simulink model "PILnewH"  (R2021a)
settings: Solver=FixedStepAuto  StartTime=0.0  StopTime=41.24  FixedStep=0.001  RelTol=1e-3  EnableMultiTasking=on
values from neighbouring files (symbols this model uses):
  den_lpf_d = den_lpf20    [Mainframe_init.m]    (also in load_autopilot.m)
  Emulated_FCC_IO_Delay = 7    [Mainframe_init.m]
  Enable_Gyros = 0    [Mainframe_init.m]
  Enable_INS = 0    [Mainframe_init.m]
  num_lpf_d = num_lpf20    [Mainframe_init.m]    (also in load_autopilot.m)
undefined symbols (not defined in the file or in its folder): act_dmp, act_omega, Actuator, Aerodynamics, aMode, Autopilot, AUX, c_b_WGS, c_be, c_flat, c_grav, c_h_geop0, c_h_geope, c_pa0, c_pe, c_r0, c_rot, c_rsma, c_Tmp0, d_siB_0, d_siB_max, d_siB_min, dd_siB_max, dd_siB_min, dev, DiscIntNeverNeededParam, e_pa, e_Tmp, Earth, fin_maxrate, flag_I_act_switch, flag_I_aero_switch, flag_I_flat, flag_I_gravity_switch, flag_I_rot, hcr, HIL_Data, JMMM_0, JMMM_e, JSPB_e, lat_0, lon_0, Mass_Props, mB_0, mM_0, mM_e, National_Instruments, pBII_0, PCIe, pMPB, pNPB, propellant_kg, prp_FBPB, prp_mdot, prp_T, pSPB, pwm_output1, qEG_0, qIB_0, qIE_0 ... (+29)
libraries: simulink x31, simulink_extras x24, aerolibcommonsys x4, px4lib x2, custom_blocks x1, pil_lib x1, aerolibtransform2 x1, sldrtlib x1, aerolibnav x1
(part 5 of 15)

== system PILnewH/Non-linear Flight Dynamic Model/GRM_Airframe/motion_kinematics/calc_motion_kinematics/earth_rotation ==
  lat : Inport
  lon : Inport  Port=2
  Gain : Gain
  Gain1 : Gain
  earth_rotation_rate : Subsystem
  quaternion_integration : Subsystem
  quaternion_integration1 : Subsystem
  transport_rate : Subsystem
  wIEE : Outport  VectorParamsAs1DForOutWhenUnconnected=off
  TIE : Outport  Port=2  VectorParamsAs1DForOutWhenUnconnected=off
  qIE : Outport  Port=3  VectorParamsAs1DForOutWhenUnconnected=off
  qEG : Outport  Port=4  VectorParamsAs1DForOutWhenUnconnected=off
  TEG : Outport  Port=5  VectorParamsAs1DForOutWhenUnconnected=off
  wEGG : Outport  Port=6  VectorParamsAs1DForOutWhenUnconnected=off
  wires:
  earth_rotation_rate/1(wIEE) -> wIEE/1, Gain/1
  Gain/1 -> quaternion_integration/1(wEIE)  "wEIE"
  quaternion_integration/1(qIE) -> qIE/1
  quaternion_integration/2(TIE) -> TIE/1
  lat/1 -> transport_rate/1(lat)
  lon/1 -> transport_rate/2(lon)
  transport_rate/1(wEGG) -> wEGG/1, Gain1/1
  Gain1/1 -> quaternion_integration1/1(wGEG)  "wGEG"
  quaternion_integration1/1(qEG) -> qEG/1
  quaternion_integration1/2(TEG) -> TEG/1

== system PILnewH/Non-linear Flight Dynamic Model/GRM_Airframe/propulsion/prp_uncertainty/3_rot_mat ==
  wi1 : Inport
  wi2 : Inport  Port=2
  wi3 : Inport  Port=3
  1. Rotation x-Achse : Subsystem
  1. Rotation y-Achse : Subsystem
  1. Rotation z-Achse : Subsystem
  2. Rotation x-Achse : Subsystem
  2. Rotation y-Achse : Subsystem
  2. Rotation z-Achse : Subsystem
  3. Rotation : Product  Inputs=***  Multiplication=Matrix(*)
  3. Rotation x-Achse : Subsystem
  3. Rotation y-Achse : Subsystem
  3. Rotation z-Achse : Subsystem
  Constant : Constant  Value=rot_1
  Constant1 : Constant  Value=rot_2
  Constant2 : Constant  Value=rot_3
  Multiport Switch : MultiPortSwitch
  Multiport Switch1 : MultiPortSwitch
  Multiport Switch2 : MultiPortSwitch
  T12 : Outport  VectorParamsAs1DForOutWhenUnconnected=off
  wires:
  Multiport Switch2/1 -> 3. Rotation/1
  Multiport Switch1/1 -> 3. Rotation/2
  Multiport Switch/1 -> 3. Rotation/3
  wi3/1 -> 3. Rotation x-Achse/1(alpha3), 3. Rotation z-Achse/1(alpha3), 3. Rotation y-Achse/1(alpha3)
  wi1/1 -> 1. Rotation z-Achse/1(alpha1), 1. Rotation y-Achse/1(alpha1), 1. Rotation x-Achse/1(alpha1)
  wi2/1 -> 2. Rotation z-Achse/1(alpha2), 2. Rotation y-Achse/1(alpha2), 2. Rotation x-Achse/1(alpha2)
  3. Rotation z-Achse/1(3Rot_Matrix_z) -> Multiport Switch2/4
  Constant/1 -> Multiport Switch/1
  1. Rotation x-Achse/1(1Rot_Matrix_x) -> Multiport Switch/2
  Constant1/1 -> Multiport Switch1/1
  1. Rotation y-Achse/1(1Rot_Matrix_y) -> Multiport Switch/3
  1. Rotation z-Achse/1(1Rot_Matrix_z) -> Multiport Switch/4
  Constant2/1 -> Multiport Switch2/1
  3. Rotation/1 -> T12/1  "T12"
  2. Rotation x-Achse/1(2Rot_Matrix_x) -> Multiport Switch1/2
  2. Rotation y-Achse/1(2Rot_Matrix_y) -> Multiport Switch1/3
  2. Rotation z-Achse/1(2Rot_Matrix_z) -> Multiport Switch1/4
  3. Rotation y-Achse/1(3Rot_Matrix_y) -> Multiport Switch2/3
  3. Rotation x-Achse/1(3Rot_Matrix_x) -> Multiport Switch2/2

== system PILnewH/Non-linear Flight Dynamic Model/GRM_Airframe/propulsion/prp_uncertainty/cross_product ==
  note: Outputs [size]:
      |
      | r1 x r2  [3x1]
  note: Inputs [size]:
      |
      | r1 [3x1]
      | r2 [3x1]
  r1 : Inport
  r2 : Inport  Port=2
  Demux2 : Demux  Outputs=[1;1;1]
      settings: DisplayOption=none
  Demux3 : Demux  Outputs=[1;1;1]
      settings: DisplayOption=none
  Product{2..7} (6 alike) : Product  InputSameDT=on  RndMeth=Zero  SaturateOnIntegerOverflow=on  OutDataTypeStr=Inherit: Same as first input
  Sum : Sum  Inputs=+-  InputSameDT=on  SaturateOnIntegerOverflow=on  OutDataTypeStr=Inherit: Same as first input
  Sum1 : Sum  Inputs=+-  InputSameDT=on  SaturateOnIntegerOverflow=on  OutDataTypeStr=Inherit: Same as first input
  Sum2 : Sum  Inputs=+-  InputSameDT=on  SaturateOnIntegerOverflow=on  OutDataTypeStr=Inherit: Same as first input
  Vector Concatenate : Concatenate  NumInputs=3  Mode=Multidimensional array
  r1_x_r2 : Outport  PortDimensions=[3,1]  VectorParamsAs1DForOutWhenUnconnected=off
  wires:
  Demux2/2 -> Product2/1, Product7/1
  Demux3/3 -> Product5/2, Product2/2
  Demux3/2 -> Product6/2, Product3/2
  Demux2/3 -> Product3/1, Product4/1
  Demux3/1 -> Product7/2, Product4/2
  Demux2/1 -> Product6/1, Product5/1
  Product2/1 -> Sum/1
  Product3/1 -> Sum/2
  Product4/1 -> Sum1/1
  Product5/1 -> Sum1/2
  Product6/1 -> Sum2/1
  Product7/1 -> Sum2/2
  Sum/1 -> Vector Concatenate/1
  Sum1/1 -> Vector Concatenate/2
  Sum2/1 -> Vector Concatenate/3
  r1/1 -> Demux2/1
  r2/1 -> Demux3/1
  Vector Concatenate/1 -> r1_x_r2/1

== system PILnewH/Non-linear Flight Dynamic Model/GRM_Airframe/rb_eom/calc_bus_flight_dyn_bus_entries/Subsystem2 ==
  TIE : Inport
  pBII : Inport  Port=2
  Constant : Constant  Value=lon_0
  Constant1 : Constant  Value=flag_I_flat
  Constant2 : Constant  Value=lat_0
  Demux : Demux  Outputs=3
  Demux1 : Demux  Outputs=3
  Gain : Gain  Gain=-1
  Math Function : Math  Operator=transpose  SignedPower=on  SaturateOnIntegerOverflow=on
  Product : Product  Multiplication=Matrix(*)
  Switch : Switch  Criteria=u2 > Threshold
  Terminator : Terminator
  Terminator1 : Terminator
  Vector Concatenate : Concatenate  NumInputs=3
  Vector Concatenate1 : Concatenate  NumInputs=3
  trafo_E_to_geodetic : Subsystem  mask(Transformation der ECEF Position in geodätische Größen){}
      mask help: Dieser Block transformiert die Position im ECEF KOS in die geodätische Länge, Breite und Höhe
      mask init:
      | [c_mue, c_rsma, c_flat] = init_transformations_earth;
      mask Help:
      | Name:
      | 
      |     trafo_E_to_geodetic
      | 
      | Beschreibung:
      | 
      |     Dieser Block transformiert die Position im ECEF KOS in die geodätische
      |     Länge, Breite und Höhe.
      | 
      | Inputs   [size]  [data type] [unit]:
      | 
      |     pBEE    [3] [double] [m]
      | 
      | Outputs  [size]  [data type] [unit]:
      | 
      |     long  [1] [double] [rad]
      |     lat   [1] [double] [rad]
      |     alt   [1] [double] [m]
      | 
      | Parameter
      | 
      |    c_rsma
      |    c_flat
  lon : Outport  VectorParamsAs1DForOutWhenUnconnected=off
  lat : Outport  Port=2  VectorParamsAs1DForOutWhenUnconnected=off
  hBE : Outport  Port=3  VectorParamsAs1DForOutWhenUnconnected=off
  wires:
  Demux1/2 -> lat/1  "lat"
  pBII/1 -> Demux/1, Product/2
  Product/1 -> trafo_E_to_geodetic/1(pBEE)  "pBEE"
  Demux1/1 -> lon/1  "lon"
  Demux1/3 -> hBE/1  "hBE"
  trafo_E_to_geodetic/1(lon) -> Vector Concatenate/1  "lon"
  trafo_E_to_geodetic/2(lat) -> Vector Concatenate/2  "lat"
  trafo_E_to_geodetic/3(alt) -> Vector Concatenate/3  "alt"
  Demux/1 -> Terminator/1
  Demux/2 -> Terminator1/1
  Demux/3 -> Gain/1
  Gain/1 -> Vector Concatenate1/3
  Constant/1 -> Vector Concatenate1/1
  Constant2/1 -> Vector Concatenate1/2
  Vector Concatenate/1 -> Switch/3
  Constant1/1 -> Switch/2
  Vector Concatenate1/1 -> Switch/1
  Switch/1 -> Demux1/1
  TIE/1 -> Math Function/1
  Math Function/1 -> Product/1  "TEI"

== system PILnewH/Non-linear Flight Dynamic Model/GRM_Airframe/rb_eom/calc_bus_flight_dyn_bus_entries/q12_from_T12 ==
  note: Outputs [size]:
      |
      | quaternion q12 [4x1]
  note: Inputs [size]:
      |
      | direction cosine matrix T12 [3x3]
  T12 : Inport  PortDimensions=[3 3]
  Case 0 : Subsystem
  Case 1 : Subsystem
  Case 2 : Subsystem
  Case 3 : Subsystem
  Constant : Constant
  Constant1 : Constant  Value=-1
  Display{,1..3} (4 alike) : Display
  Merge : Merge  Inputs=4
  Product4 : Product
  Selector : Selector  IndexMode=Zero-based  InputPortWidth=4  IndexOptions=Index vector (dialog)  Indices=3  OutputSizes=1
  Switch : Switch
  dcm11 : Selector  NumberOfDimensions=2  IndexMode=Zero-based  InputPortWidth=3  IndexOptions=Index vector (dialog),Index vector (dialog)  Indices=0,0  OutputSizes=1,1
  dcm22 : Selector  NumberOfDimensions=2  IndexMode=Zero-based  InputPortWidth=3  IndexOptions=Index vector (dialog),Index vector (dialog)  Indices=1,1  OutputSizes=1,1
  dcm33 : Selector  NumberOfDimensions=2  IndexMode=Zero-based  InputPortWidth=3  IndexOptions=Index vector (dialog),Index vector (dialog)  Indices=2,2  OutputSizes=1,1
  normalize_quaternion : Subsystem
      mask help: normalize a quaternion
      mask Help:
      | Name:
      | 
      |     normalize_quaternion
      | 
      | Description:
      | 
      |     This block normalizes the quaternion q21. It should be used as a
      |     safety measure when computing quaternions.
      | 
      | Inputs  [size] [data type] [unit]:
      | 
      |     attitude quaternion q21  [4] [double] [-]
      | 
      | Outputs  [size] [data type] [unit]:
      | 
      |     normalized attitude quaternion q21  [4] [double] [-]
      mask Display: disp (' norm(q)')
  q_R^0(R) : Subsystem  TreatAsAtomicUnit=on
  q_R^1(R) : Subsystem  TreatAsAtomicUnit=on
  q_R^2(R) : Subsystem  TreatAsAtomicUnit=on
  q_R^3(R) : Subsystem  TreatAsAtomicUnit=on
  q12 : Outport  PortDimensions=[4 1]  VectorParamsAs1DForOutWhenUnconnected=off
  wires:
  Constant1/1 -> Switch/3
  Switch/1 -> Product4/2
  Selector/1 -> Switch/2
  normalize_quaternion/1(q_normalized) -> Selector/1, Product4/1
  Constant/1 -> Switch/1
  Product4/1 -> q12/1
  Merge/1 -> normalize_quaternion/1(q)
  q_R^1(R)/1(q_R^1(R)) -> Merge/2
  q_R^2(R)/1(q_R^2(R)) -> Merge/3
  q_R^3(R)/1(q_R^3(R)) -> Merge/4
  q_R^0(R)/1(q_R^0(R)) -> Merge/1
  Case 3/1(q_R^3(R)) -> q_R^3(R)/Enable, Display3/1
  Case 2/1(q_R^2(R)) -> q_R^2(R)/Enable, Display2/1
  T12/1 -> q_R^0(R)/1(DCM), q_R^1(R)/1(DCM), q_R^2(R)/1(DCM), q_R^3(R)/1(DCM), dcm33/1, dcm22/1, dcm11/1
  Case 1/1(q_R^1(R)) -> q_R^1(R)/Enable, Display1/1
  Case 0/1(q_R^0(R)) -> q_R^0(R)/Enable, Display/1
  dcm33/1 -> Case 3/3(dcm33), Case 2/3(dcm33), Case 1/3(dcm33), Case 0/3(dcm33)  "dcm33"
  dcm22/1 -> Case 3/2(dcm22), Case 2/2(dcm22), Case 1/2(dcm22), Case 0/2(dcm22)  "dcm22"
  dcm11/1 -> Case 3/1(dcm11), Case 2/1(dcm11), Case 1/1(dcm11), Case 0/1(dcm11)  "dcm11"

== system PILnewH/Non-linear Flight Dynamic Model/GRM_Airframe/rb_eom/calc_bus_flight_dyn_bus_entries/quaternion_to_euler_angles ==
  note: Inputs [size]:
      |
      | quaternion [4]
  note: Outputs [size]:
      |
      | roll angle [1]
      | pitch angle [1]
      | yaw angle [1]
  note: Um numerische Probleme zu
      | vermeiden, wird hier eine Saturiierung
      | benutzt.
  q : Inport  PortDimensions=4
  Add : Sum
  Add1 : Sum  Inputs=+--
  Add2 : Sum  Inputs=+-
  Add3 : Sum
  Add4 : Sum  Inputs=+--
  Complex to Real-Imag : ComplexToRealImag  Output=Real
  Constant : Constant  Value=0.5
  Constant1 : Constant  Value=0.5
  Demux : Demux
  Gain : Gain  Gain=2
  Product{,1..9} (10 alike) : Product
  Saturation : Saturate  UpperLimit=1  LowerLimit=-1
      settings: AttributesFormatString=|
      | %<UpperLimit>
      | %<LowerLimit>
  Trigonometric Function : Trigonometry  Operator=atan2
  Trigonometric Function1 : Trigonometry  Operator=asin
  Trigonometric Function2 : Trigonometry  Operator=atan2
  Vector Concatenate : Concatenate  NumInputs=3
  eulx : Outport  VectorParamsAs1DForOutWhenUnconnected=off
  wires:
  Saturation/1 -> Trigonometric Function1/1
  Gain/1 -> Saturation/1
  Demux/3 -> Product5/2, Product1/2, Product7/1, Product9/1, Product9/2  "3"
  Constant1/1 -> Add4/1
  Product8/1 -> Add4/2
  Product9/1 -> Add4/3
  Constant/1 -> Add1/1
  Demux/2 -> Product6/2, Product8/1, Product8/2, Product1/1, Product3/1, Product3/2, Product4/1  "2"
  Demux/1 -> Product5/1, Product6/1, Product/1, Product2/1, Product2/2  "1"
  Demux/4 -> Product/2, Product4/2, Product7/2  "4"
  q/1 -> Demux/1
  Add1/1 -> Trigonometric Function/2
  Add2/1 -> Gain/1
  Add4/1 -> Trigonometric Function2/2
  Add3/1 -> Trigonometric Function2/1
  Product6/1 -> Add3/1
  Product7/1 -> Add3/2
  Product4/1 -> Add2/1
  Product5/1 -> Add2/2
  Product2/1 -> Add1/2
  Product3/1 -> Add1/3
  Product/1 -> Add/1
  Product1/1 -> Add/2
  Add/1 -> Trigonometric Function/1
  Trigonometric Function/1 -> Vector Concatenate/1
  Trigonometric Function1/1 -> Vector Concatenate/2
  Trigonometric Function2/1 -> Vector Concatenate/3
  Complex to Real-Imag/1 -> eulx/1
  Vector Concatenate/1 -> Complex to Real-Imag/1

== system PILnewH/Non-linear Flight Dynamic Model/GRM_Airframe/rb_eom/calc_bus_flight_dyn_bus_entries/quaternion_to_euler_angles1 ==
  note: Um numerische Probleme zu
      | vermeiden, wird hier eine Saturiierung
      | benutzt.
  note: Outputs [size]:
      |
      | roll angle [1]
      | pitch angle [1]
      | yaw angle [1]
  note: Inputs [size]:
      |
      | quaternion [4]
  q : Inport  PortDimensions=4
  Add : Sum
  Add1 : Sum  Inputs=+--
  Add2 : Sum  Inputs=+-
  Add3 : Sum
  Add4 : Sum  Inputs=+--
  Complex to Real-Imag : ComplexToRealImag  Output=Real
  Constant : Constant  Value=0.5
  Constant1 : Constant  Value=0.5
  Demux : Demux
  Gain : Gain  Gain=2
  Product{,1..9} (10 alike) : Product
  Saturation : Saturate  UpperLimit=1  LowerLimit=-1
      settings: AttributesFormatString=|
      | %<UpperLimit>
      | %<LowerLimit>
  Trigonometric Function : Trigonometry  Operator=atan2
  Trigonometric Function1 : Trigonometry  Operator=asin
  Trigonometric Function2 : Trigonometry  Operator=atan2
  Vector Concatenate : Concatenate  NumInputs=3
  eulx : Outport  VectorParamsAs1DForOutWhenUnconnected=off
  wires:
  Vector Concatenate/1 -> Complex to Real-Imag/1
  Complex to Real-Imag/1 -> eulx/1
  Trigonometric Function2/1 -> Vector Concatenate/3
  Trigonometric Function1/1 -> Vector Concatenate/2
  Trigonometric Function/1 -> Vector Concatenate/1
  Add/1 -> Trigonometric Function/1
  Product1/1 -> Add/2
  Product/1 -> Add/1
  Product3/1 -> Add1/3
  Product2/1 -> Add1/2
  Product5/1 -> Add2/2
  Product4/1 -> Add2/1
  Product7/1 -> Add3/2
  Product6/1 -> Add3/1
  Add3/1 -> Trigonometric Function2/1
  Add4/1 -> Trigonometric Function2/2
  Add2/1 -> Gain/1
  Add1/1 -> Trigonometric Function/2
  q/1 -> Demux/1
  Demux/4 -> Product7/2, Product4/2, Product/2  "4"
  Demux/1 -> Product2/2, Product2/1, Product/1, Product6/1, Product5/1  "1"
  Demux/2 -> Product4/1, Product3/2, Product3/1, Product1/1, Product8/2, Product8/1, Product6/2  "2"
  Constant/1 -> Add1/1
  Product9/1 -> Add4/3
  Product8/1 -> Add4/2
  Constant1/1 -> Add4/1
  Demux/3 -> Product9/2, Product9/1, Product7/1, Product1/2, Product5/2  "3"
  Gain/1 -> Saturation/1
  Saturation/1 -> Trigonometric Function1/1

== system PILnewH/Non-linear Flight Dynamic Model/GRM_Airframe/rb_eom/eom_6dof/Rigid_Body_EOM_6_DOF ==
  FBTX : Inport  PortDimensions=[3,1]
  MBTB : Inport  Port=2  PortDimensions=[3,1]
  mB : Inport  Port=3  PortDimensions=[1]
  x0 : Inport  Port=4
  JBB : Inport  Port=5  PortDimensions=[3,3]
  d_JBB : Inport  Port=6  PortDimensions=[3,3]
  Bus Selector : BusSelector  OutputSignals=qIB,vBII,wBIB
  Constant : Constant  Value=flag_Kraft
  Integration : Subsystem
  Math Function2 : Math  Operator=transpose  SignedPower=on  SaturateOnIntegerOverflow=on
  Product2 : Product  Multiplication=Matrix(*)
  Switch : Switch  Criteria=u2 > Threshold  Threshold=1
  T12_from_q12 : Subsystem
      mask help: Transforms a quaternion into a Direction Cosine Matrix
      mask Help:
      | Name:
      | 
      |     T12_from_q12
      | 
      | Description:
      | 
      |     This block implements the transformation of a quaternion into the
      |     corresponding direction cosine matrix DCM.
      | 
      | Inputs  [size] [data type] [unit]:
      | 
      |     quaternion q12 [4] [double] [-]
      | 
      | Outputs  [size] [data type] [unit]:
      | 
      |     direction cosine matrix T12  [3x3] [double] [-]
      mask Display:
      | %port_label('input', 1, 'q12')
      | %port_label('output', 1, 'T12')
      | disp('q \rightarrow DCM','texmode','on')
  rb_eom_6dof : Subsystem
  rb_eom : Outport  VectorParamsAs1DForOutWhenUnconnected=off
  wires:
  rb_eom_6dof/4(d_wBIB) -> Integration/4(d_wBIB)  "d_wBIB"
  JBB/1 -> rb_eom_6dof/3(JBB)
  d_JBB/1 -> rb_eom_6dof/5(d_JBB)
  mB/1 -> rb_eom_6dof/2(mB)
  MBTB/1 -> rb_eom_6dof/4(MBTB)
  Switch/1 -> rb_eom_6dof/1(FBTB)
  Constant/1 -> Switch/2
  Product2/1 -> Switch/3
  FBTX/1 -> Product2/2, Switch/1
  Math Function2/1 -> Product2/1
  T12_from_q12/1(T12) -> Math Function2/1
  Bus Selector/2 -> rb_eom_6dof/7(vBII)  "<vBII>"
  x0/1 -> Integration/5(x0)
  Bus Selector/1 -> rb_eom_6dof/6(qIB), T12_from_q12/1(q12)  "<qIB>"
  Bus Selector/3 -> rb_eom_6dof/8(wBIB)  "<wBIB>"
  rb_eom_6dof/1(d_pBII) -> Integration/1(d_pBII)  "d_pBII"
  rb_eom_6dof/2(d_vBII) -> Integration/2(d_vBII)  "d_vBII"
  rb_eom_6dof/3(d_qIB) -> Integration/3(d_qIB)  "d_qIB"
  Integration/1(eom) -> Bus Selector/1, rb_eom/1

== system PILnewH/Non-linear Flight Dynamic Model/GRM_Airframe/stream_flow/calc_stream_flow/Subsystem1 ==
  vBEB : Inport
  wBIB : Inport  Port=2
  rho : Inport  Port=3
  sos : Inport  Port=4
  AoA_Sideslip_Alphatot_Phi : Subsystem
      mask help:
      | Aus den Komponenten der Geschwindigkeit im ECEF-System, dargestellt im Body-System vBEB
      | werden Anstellwinkel (alpha), Schiebewinkel (beta), totaler Anstellwinkel (alpha_T) sowie Rollwinkel (phi) berechnet.
      | Die Ausgabe erfolgt als Bus in [rad]
      mask Help:
      | Name:
      | 
      |    AoA_sideslip_alphatot_phi
      | 
      | Beschreibung:
      | 
      |   Dieser Block berechnet Anstellwinkel, Schiebewinkel, totalen Anstellwinkel und Rollwinkel in [rad]
      |   aus der Geschwindigkeit vBEB (ECEF-System dargestellt in Body-Koordinaten)
      | 
      | Inputs   [dimension]  [data type] [unit]:
      | 
      |     vBEB    [3] [double] [m/s]
      | 
      | Outputs  [dimension]  [data type] [unit]:
      | 
      | aero_angle_bus [4] [bus] [-]
      |     alpha     [1] [double] [rad]
      |     beta       [1] [double] [rad]
      |     alpha_T [1] [double] [rad]
      |     phi         [1] [double] [rad]
      mask Display:
      | %port_label('input', 1, 'vBEB')
      | %port_label('output', 1, 'aero_angles')
      | disp('vBEB \rightarrow \alpha \beta \alpha_T \phi','texmode','on')
  Bus Selector : BusSelector  OutputSignals=al,be,th,fi
  Constant : Constant  Value=0.5
  Divide : Product  Inputs=*/
  Math Function1 : Math  Operator=square  SignedPower=on  SaturateOnIntegerOverflow=on
  Product1 : Product  Inputs=3
  calc_nondimensional_rates : Subsystem
  norm_of_vector : Subsystem
      mask help: computes the norm of a vector
      mask Help:
      | Name:
      | 
      |     norm_of_vector
      | 
      | Description:
      | 
      |     This block computes the L2-norm (length) of a vector.
      | 
      | Inputs  [size] [data type] [unit]:
      | 
      |     vector  [3] [double] [-]
      | 
      | Outputs  [size] [data type] [unit]:
      | 
      |     norm of vector  [1] [double] [-]
      mask Display: disp (' norm(r) ')
  al : Outport  VectorParamsAs1DForOutWhenUnconnected=off
  be : Outport  Port=2  VectorParamsAs1DForOutWhenUnconnected=off
  qdynB : Outport  Port=3  VectorParamsAs1DForOutWhenUnconnected=off
  MaB : Outport  Port=4  VectorParamsAs1DForOutWhenUnconnected=off
  a_vB : Outport  Port=5  VectorParamsAs1DForOutWhenUnconnected=off
  wBIB_star : Outport  Port=6  VectorParamsAs1DForOutWhenUnconnected=off
  th : Outport  Port=7  VectorParamsAs1DForOutWhenUnconnected=off
  fi : Outport  Port=8  VectorParamsAs1DForOutWhenUnconnected=off
  wires:
  sos/1 -> Divide/2
  AoA_Sideslip_Alphatot_Phi/1(aero_angles) -> Bus Selector/1
  vBEB/1 -> norm_of_vector/1(vector), AoA_Sideslip_Alphatot_Phi/1(vBEB)
  norm_of_vector/1(norm_of_vector) -> Math Function1/1, calc_nondimensional_rates/1(a_vB), a_vB/1, Divide/1  "a_vB"
  Product1/1 -> qdynB/1  "qdynB"
  Math Function1/1 -> Product1/1
  Constant/1 -> Product1/2
  Divide/1 -> MaB/1  "MaB"
  Bus Selector/2 -> be/1  "<be>"
  rho/1 -> Product1/3
  Bus Selector/1 -> al/1  "<al>"
  wBIB/1 -> calc_nondimensional_rates/2(wBIB)
  calc_nondimensional_rates/1(wBIB_star) -> wBIB_star/1
  Bus Selector/3 -> th/1  "<th>"
  Bus Selector/4 -> fi/1  "<fi>"

== system PILnewH/Non-linear Flight Dynamic Model/GRM_Airframe/stream_flow/calc_stream_flow/velocity_vector_transformation ==
  wIEE : Inport
  TIE : Inport  Port=2
  vBII : Inport  Port=3
  pBII : Inport  Port=4
  Add : Sum  Inputs=+-
  Product : Product  Multiplication=Matrix(*)
  cross_product : Subsystem
      mask help: cross product r3 = r1 x r2
      mask Help:
      | Name:
      | 
      |     cross_product
      | 
      | Description:
      | 
      |     This block implements the cross product r3 = r1 x r2.
      | 
      | Inputs  [size] [data type] [unit]:
      | 
      |     vector 1  [3] [double] [-]
      |     vector 2  [3] [double] [-]
      | 
      | Outputs  [size] [data type] [unit]:
      | 
      |     resulting vector  [3] [double] [-]
      mask Display: disp(' r3 = r1 x r2')
  vBEI : Outport  VectorParamsAs1DForOutWhenUnconnected=off
  wires:
  TIE/1 -> Product/1
  wIEE/1 -> Product/2
  Product/1 -> cross_product/1(r1)  "wIEI"
  pBII/1 -> cross_product/2(r2)
  cross_product/1(r1_x_r2) -> Add/2  "de_vBEI"
  vBII/1 -> Add/1
  Add/1 -> vBEI/1  "vBEI"

== system PILnewH/Non-linear Flight Dynamic Model/GRM_Airframe/weight_and_balance/moi/JMMM_linear_interpolation ==
  mM : Inport
  Constant16 : Constant  Value=JMMM_0
  Constant17 : Constant  Value=JMMM_e
  Constant18 : Constant  Value=mM_0
  Constant19 : Constant  Value=mM_e
  Constant20 : Constant  Value=mM_0
  Constant21 : Constant  Value=JMMM_0
  Divide : Product  Inputs=**/
  Subtract : Sum  Inputs=+-
  Subtract4 : Sum  Inputs=+-
  Subtract5 : Sum  Inputs=+-
  Subtract6 : Sum
  JMMM : Outport  VectorParamsAs1DForOutWhenUnconnected=off
  wires:
  mM/1 -> Subtract5/1
  Subtract5/1 -> Divide/1
  Constant20/1 -> Subtract5/2
  Constant19/1 -> Subtract4/1
  Constant18/1 -> Subtract4/2
  Constant17/1 -> Subtract/1
  Constant16/1 -> Subtract/2
  Subtract/1 -> Divide/2
  Subtract4/1 -> Divide/3
  Subtract6/1 -> JMMM/1  "JMMM"
  Constant21/1 -> Subtract6/1
  Divide/1 -> Subtract6/2

== system PILnewH/Non-linear Flight Dynamic Model/GRM_Airframe/weight_and_balance/moi/moi_coordinate_transformation ==
  JMMM : Inport
  3_rot_mat : Subsystem  mask(Rotation um 1, 2 oder 3 Achsen){rot_1=Rotation um z-Achse, rot_2=Rotation um y-Achse, rot_3=Rotation um x-Achse}
      mask prompts: rot_1 "1. Rotation"; rot_2 "2. Rotation"; rot_3 "3. Rotation"
      mask help:
      | Dieser Block liefert die Rotationsmatrix T12 für den Fall zurück, dass sich das Ziel-Koordinatensystem (1) durch Drehungen um 1, 2 oder 3 Achsen gegenüber dem Ausgangskoordinatensystem (2) beschreiben lässt (passive Drehung).
      |
      | Die Anzahl der Rotation sowie die Reihenfolge ist frei einstellbar.
      |
      | Die Rotationswinkel haben die Einheit [rad].
      mask TypeOptions rot_1: Rotation um x-Achse | Rotation um y-Achse | Rotation um z-Achse
      mask TypeOptions rot_2: Rotation um x-Achse | Rotation um y-Achse | Rotation um z-Achse
      mask TypeOptions rot_3: Rotation um x-Achse | Rotation um y-Achse | Rotation um z-Achse
  Math Function : Math  Operator=transpose  SignedPower=on  SaturateOnIntegerOverflow=on
  Matrix Multiply : Product  Multiplication=Matrix(*)
  Matrix Multiply1 : Product  Multiplication=Matrix(*)
  Thrust_rot_z : Constant  Value=unc_prp_z
  thrust_rot_x : Constant  Value=unc_prp_x
  thrust_rot_y : Constant  Value=unc_prp_y
  JMMB : Outport  VectorParamsAs1DForOutWhenUnconnected=off
  wires:
  Math Function/1 -> Matrix Multiply1/2
  Matrix Multiply/1 -> Matrix Multiply1/1
  JMMM/1 -> Matrix Multiply/2
  3_rot_mat/1(T12) -> Math Function/1, Matrix Multiply/1
  Matrix Multiply1/1 -> JMMB/1  "JMMB"
  thrust_rot_y/1 -> 3_rot_mat/2(wi2)
  thrust_rot_x/1 -> 3_rot_mat/3(wi3)
  Thrust_rot_z/1 -> 3_rot_mat/1(wi1)

== system PILnewH/Non-linear Flight Dynamic Model/GRM_Airframe/weight_and_balance/moi/moi_uncertainty ==
  JBBB_c : Inport
  Add7 : Sum
  Constant16 : Constant  Value=[unc_moi_Jxx,0,0;0,unc_moi_Jyy,0;0,0,unc_moi_Jzz]
  JBBB : Outport  VectorParamsAs1DForOutWhenUnconnected=off
  wires:
  Add7/1 -> JBBB/1  "JBBB"
  JBBB_c/1 -> Add7/1
  Constant16/1 -> Add7/2

== system PILnewH/Non-linear Flight Dynamic Model/GRM_Airframe/weight_and_balance/moi/steiners_theorem_missile ==
  pBPB : Inport
  Constant : Constant  Value=mB_0
  Constant17 : Constant  Value=pSPB
  Product : Product
  Subtract : Sum  Inputs=+-
  create_deviation_matrix : Subsystem
  J_deviation : Outport  VectorParamsAs1DForOutWhenUnconnected=off
  wires:
  pBPB/1 -> Subtract/1
  Product/1 -> J_deviation/1
  create_deviation_matrix/1(T_deviation) -> Product/2
  Constant17/1 -> Subtract/2
  Subtract/1 -> create_deviation_matrix/1(pBXB)  "pB0B"
  Constant/1 -> Product/1

== system PILnewH/Non-linear Flight Dynamic Model/GRM_Airframe/weight_and_balance/moi/steiners_theorem_motor ==
  pBPB : Inport
  mM : Inport  Port=2
  Constant16 : Constant  Value=pMPB
  Product : Product
  Subtract4 : Sum  Inputs=+-
  create_deviation_matrix1 : Subsystem
  JM_deviation : Outport  VectorParamsAs1DForOutWhenUnconnected=off
  wires:
  Product/1 -> JM_deviation/1
  pBPB/1 -> Subtract4/1
  create_deviation_matrix1/1(T_deviation) -> Product/1
  Constant16/1 -> Subtract4/2
  Subtract4/1 -> create_deviation_matrix1/1(pBXB)  "pBMB"
  mM/1 -> Product/2

== system PILnewH/Non-linear Flight Dynamic Model/Subsystem1/Extract States/Assemble_States_Bus1/Rotation Angles to Quaternions ==
  "R1, R2, R3" : Inport  Unit=rad
  1/2 : Gain  Gain=0.5  SaturateOnIntegerOverflow=on  OutDataTypeStr=Inherit: Same as input  ParamDataTypeStr=Inherit: Same as input
  Mux1 : Mux  Inputs=2
  Mux2 : Mux
  q0 : Fcn  Expr=u(4)*u(5)*u(6) + u(1)*u(2)*u(3)
  q1 : Fcn  Expr=u(4)*u(5)*u(3) - u(1)*u(2)*u(6)
  q2 : Fcn  Expr=u(4)*u(2)*u(6) + u(1)*u(5)*u(3)
  q3 : Fcn  Expr=u(1)*u(5)*u(6) - u(4)*u(2)*u(3)
  sincos : Trigonometry  Operator=sincos
  Quat : Outport  Unit=1  InitialOutput=0  VectorParamsAs1DForOutWhenUnconnected=off
  wires:
  q0/1 -> Mux2/1
  Mux2/1 -> Quat/1
  q3/1 -> Mux2/4
  q2/1 -> Mux2/3
  q1/1 -> Mux2/2
  Mux1/1 -> q3/1, q2/1, q1/1, q0/1
  sincos/2 -> Mux1/2
  sincos/1 -> Mux1/1
  1/2/1 -> sincos/1
  "R1, R2, R3"/1 -> 1/2/1

== system PILnewH/Non-linear Flight Dynamic Model/Subsystem1/Extract States/Assemble_States_Bus1/Three-axis Inertial Measurement Unit3 ==
  A_b : Inport  Unit=m/s^2
  w : Inport  Port=2  Unit=rad/s
  w_dot : Inport  Port=3  Unit=rad/s^2
  CG : Inport  Port=4  Unit=m
  g : Inport  Port=5  Unit=m/s^2
  Acceleration Conversion : Subsystem
  Disallow CGS : UnitConfiguration  UnitSystemsStr=English,SI,SI (extended)  AllowAllUnitSystems=off
  Three-axis Accelerometer : Subsystem  mask(Three-axis Accelerometer){units=Metric (MKS), acc=imu, gtype=on, dtype_a=on, w_a=w_a, z_a=z_a, a_sf_cc=a_sf_cc, a_bias=a_bias, a_Ts=i_Ts, a_rand=on, a_seeds=i_seeds(1:3), a_pow=i_pow(1:3), a_sat=a_sat}
      mask prompts: units "aeroblks:aeroblknav:blockThreeaxisAccelerometerParamUnits"; acc "aeroblks:aeroblknav:blockThreeaxisAccelerometerParamAccelerometerlocation"; gtype "aeroblks:aeroblknav:blockThreeaxisAccelerometerParamSubtractgravity"; dtype_a "aeroblks:aeroblknav:blockThreeaxisAccelerometerParamSecondorderdynamics"; w_a "aeroblks:aeroblknav:blockThreeaxisAccelerometerParamNaturalfrequencyradsec"; z_a "aeroblks:aeroblknav:blockThreeaxisAccelerometerParamDampingratio"; a_sf_cc "aeroblks:aeroblknav:blockThreeaxisAccelerometerParamScalefactorsandcrosscoupling"; a_bias "aeroblks:aeroblknav:blockThreeaxisAccelerometerParamMeasurementbias"; a_Ts "aeroblks:aeroblknav:blockThreeaxisAccelerometerParamUpdateratesec"; a_rand "aeroblks:aeroblknav:blockThreeaxisAccelerometerParamNoiseon"; a_seeds "aeroblks:aeroblknav:blockThreeaxisAccelerometerParamNoiseseeds"; a_pow "aeroblks:aeroblknav:blockThreeaxisAccelerometerParamNoisepower"; a_sat "aeroblks:aeroblknav:blockThreeaxisAccelerometerParamLowerandupperoutputlimits"
      mask help: aeroblks:aeroblknav:blockThreeaxisAccelerometerDesc
      mask init:
      | par = a_Ts;
      | block = gcb;
      | ports=aeroicon('aeroblkaccel','icon',par);
      | a_satl = a_sat(1:3);
      | a_sath = a_sat(4:6);
      mask Help: eval('asbhelp');
      mask TypeOptions units: aeroblks:aeroblknav:blockThreeaxisAccelerometerParamComboMetricMKS | aeroblks:aeroblknav:blockThreeaxisAccelerometerParamComboEnglish
      mask Callback gtype: aeroicon('aeroblkaccel')
      mask Callback dtype_a: aeroicon('aeroblkaccel')
      mask Callback a_rand: aeroicon('aeroblkaccel')
      mask DialogControl ParameterTabVar0 Prompt: Main
      mask DialogControl units Prompt: Units:
      mask DialogControl acc Prompt: Accelerometer location:
      mask DialogControl gtype Prompt: Subtract gravity:
      mask DialogControl dtype_a Prompt: Second-order dynamics
      mask DialogControl w_a Prompt: Natural frequency (rad/sec):
      mask DialogControl z_a Prompt: Damping ratio:
      mask DialogControl a_sf_cc Prompt: Scale factors and cross-coupling:
      mask DialogControl a_bias Prompt: Measurement bias:
      mask DialogControl a_Ts Prompt: Update rate (sec):
      mask DialogControl ParameterTabVar01 Prompt: Noise
      mask DialogControl a_rand Prompt: Noise on
      mask DialogControl a_seeds Prompt: Noise seeds:
      mask DialogControl a_pow Prompt: Noise power:
      mask DialogControl a_sat Prompt: Lower and upper output limits:
      mask Display:
      | port_label(ports(1).type,ports(1).port,ports(1).txt,'texmode','on');
      | port_label(ports(2).type,ports(2).port,ports(2).txt,'texmode','on');
      | port_label(ports(3).type,ports(3).port,ports(3).txt,'texmode','on');
      | port_label(ports(4).type,ports(4).port,ports(4).txt,'texmode','on');
      | port_label(ports(5).type,ports(5).port,ports(5).txt,'texmode','on');
      | port_label(ports(6).type,ports(6).port,ports(6).txt,'texmode','on');
  Three-axis Gyroscope : Subsystem  mask(Three-axis Gyroscope){dtype_g=on, w_g=w_g, z_g=z_g, g_sf_cc=g_sf_cc, g_bias=g_bias, g_sen=g_sens, g_Ts=i_Ts, g_rand=on, g_seeds=i_seeds(4:6), g_pow=i_pow(4:6), g_sat=g_sat}
      mask prompts: dtype_g "aeroblks:aeroblknav:blockThreeaxisGyroscopeParamSecondorderdynamics"; w_g "aeroblks:aeroblknav:blockThreeaxisGyroscopeParamNaturalfrequencyradsec"; z_g "aeroblks:aeroblknav:blockThreeaxisGyroscopeParamDampingratio"; g_sf_cc "aeroblks:aeroblknav:blockThreeaxisGyroscopeParamScalefactorsandcrosscoupling"; g_bias "aeroblks:aeroblknav:blockThreeaxisGyroscopeParamMeasurementbias"; g_sen "aeroblks:aeroblknav:blockThreeaxisGyroscopeParamGsensitivebias"; g_Ts "aeroblks:aeroblknav:blockThreeaxisGyroscopeParamUpdateratesec"; g_rand "aeroblks:aeroblknav:blockThreeaxisGyroscopeParamNoiseon"; g_seeds "aeroblks:aeroblknav:blockThreeaxisGyroscopeParamNoiseseeds"; g_pow "aeroblks:aeroblknav:blockThreeaxisGyroscopeParamNoisepower"; g_sat "aeroblks:aeroblknav:blockThreeaxisGyroscopeParamLowerandupperoutputlimits"
      mask help: aeroblks:aeroblknav:blockThreeaxisGyroscopeDesc
      mask init:
      | par = g_Ts;
      | block = gcb;
      | g_satl = g_sat(1:3);
      | g_sath = g_sat(4:6);
      | ports=aeroicon('aeroblkgyro','icon',par);
      mask Help: eval('asbhelp');
      mask Callback dtype_g: aeroicon('aeroblkgyro');
      mask Callback g_rand: aeroicon('aeroblkgyro');
      mask DialogControl ParameterTabVar0 Prompt: Main
      mask DialogControl dtype_g Prompt: Second-order dynamics
      mask DialogControl w_g Prompt: Natural frequency (rad/sec):
      mask DialogControl z_g Prompt: Damping ratio:
      mask DialogControl g_sf_cc Prompt: Scale factors and cross-coupling:
      mask DialogControl g_bias Prompt: Measurement bias:
      mask DialogControl g_sen Prompt: G-sensitive bias:
      mask DialogControl g_Ts Prompt: Update rate (sec):
      mask DialogControl ParameterTabVar01 Prompt: Noise
      mask DialogControl g_rand Prompt: Noise on
      mask DialogControl g_seeds Prompt: Noise seeds:
      mask DialogControl g_pow Prompt: Noise power:
      mask DialogControl g_sat Prompt: Lower and upper output limits:
      mask Display:
      | port_label(ports(1).type,ports(1).port,ports(1).txt,'texmode','on');
      | port_label(ports(2).type,ports(2).port,ports(2).txt,'texmode','on');
      | port_label(ports(3).type,ports(3).port,ports(3).txt,'texmode','on');
  A_meas : Outport  Unit=m/s^2  VectorParamsAs1DForOutWhenUnconnected=off
  w_meas : Outport  Port=2  Unit=rad/s  VectorParamsAs1DForOutWhenUnconnected=off
  wires:
  Three-axis Accelerometer/1(Ameas) -> A_meas/1
  Three-axis Gyroscope/1((p q r)_meas) -> w_meas/1
  A_b/1 -> Acceleration Conversion/1(acceleration), Three-axis Accelerometer/1(Ab)
  w/1 -> Three-axis Accelerometer/2(p q r), Three-axis Gyroscope/1(p q r)
  CG/1 -> Three-axis Accelerometer/4(CG)
  w_dot/1 -> Three-axis Accelerometer/3(pdot qdot rdot)
  Acceleration Conversion/1(inherit) -> Three-axis Gyroscope/2(G's)
  g/1 -> Three-axis Accelerometer/5(g)

== system PILnewH/Non-linear Flight Dynamic Model/Subsystem1/GRM_Airframe/aerodynamics/aerodynamic_via_lookup ==
  pBPB : Inport
  qdynB : Inport  Port=2
  MaB : Inport  Port=3
  alB : Inport  Port=4
  beB : Inport  Port=5
  hBE : Inport  Port=6
  wBIB_star : Inport  Port=7
  afinB : Inport  Port=8
  flag_I_prp : Inport  Port=9
  Bus Creator : BusCreator  Inputs=2
  Demux1 : Demux  Outputs=3
  Demux3 : Demux  Outputs=3
  Gain{,1..4} (5 alike) : Gain  Gain=180/pi
      settings: AttributesFormatString=%<Gain>
  Saturation1 : Saturate  UpperLimit=Aerodynamics.ulim_alpha_deg  LowerLimit=Aerodynamics.llim_alpha_deg
      settings: AttributesFormatString=|
      | %<UpperLimit>
      | %<LowerLimit>
  Saturation4 : Saturate  UpperLimit=Aerodynamics.ulim_beta_deg  LowerLimit=Aerodynamics.llim_beta_deg
      settings: AttributesFormatString=|
      | %<UpperLimit>
      | %<LowerLimit>
  Terminator : Terminator
  Terminator1 : Terminator
  calc_aero_coefficients : Subsystem
  calc_aero_for_mom : Subsystem
  aero_bus : Outport  VectorParamsAs1DForOutWhenUnconnected=off
  wires:
  MaB/1 -> Terminator1/1
  calc_aero_for_mom/1(FBAB) -> Bus Creator/1
  Bus Creator/1 -> aero_bus/1  "aero_bus"
  pBPB/1 -> calc_aero_for_mom/2(pBPB)
  flag_I_prp/1 -> Terminator/1
  hBE/1 -> calc_aero_for_mom/1(hBE)
  calc_aero_for_mom/2(MBAB) -> Bus Creator/2
  qdynB/1 -> calc_aero_for_mom/3(qdynB)
  alB/1 -> Gain3/1
  beB/1 -> Gain4/1
  wBIB_star/1 -> Demux1/1
  Demux1/1 -> calc_aero_coefficients/4(pBIB_star_rps)  "pBIB_star_rps"
  Demux1/2 -> calc_aero_coefficients/5(qBIB_star_rps)  "qBIB_star_rps"
  Demux1/3 -> calc_aero_coefficients/6(rBIB_star_rps)  "rBIB_star_rps"
  afinB/1 -> Demux3/1
  Demux3/2 -> Gain1/1  "etB"
  Demux3/1 -> Gain/1  "xiB"
  Demux3/3 -> Gain2/1  "zeB"
  Gain/1 -> calc_aero_coefficients/1(dela_deg)
  Gain1/1 -> calc_aero_coefficients/2(dele_deg)
  Gain2/1 -> calc_aero_coefficients/3(delr_deg)
  calc_aero_coefficients/1(Cx) -> calc_aero_for_mom/4(Cx)
  calc_aero_coefficients/2(Cy) -> calc_aero_for_mom/5(Cy)
  calc_aero_coefficients/3(Cz) -> calc_aero_for_mom/6(Cz)
  calc_aero_coefficients/4(Cl) -> calc_aero_for_mom/7(Cl)
  calc_aero_coefficients/5(Cm) -> calc_aero_for_mom/8(Cm)
  calc_aero_coefficients/6(Cn) -> calc_aero_for_mom/9(Cn)
  Saturation1/1 -> calc_aero_coefficients/7(alB_deg)
  Saturation4/1 -> calc_aero_coefficients/8(beB_deg)
  Gain3/1 -> Saturation1/1
  Gain4/1 -> Saturation4/1

== system PILnewH/Non-linear Flight Dynamic Model/Subsystem1/GRM_Airframe/aerodynamics/logic_base_drag ==
  env_glbl : Inport
  Bus Selector1 : BusSelector  OutputSignals=T_sim_glbl,T_sim_lnch
  Constant : Constant  Value=prp_T(end)
  MATLAB Function : MATLAB Function  TreatAsAtomicUnit=on
  Subtract : Sum  Inputs=+-
  flag_base_drag : Outport  VectorParamsAs1DForOutWhenUnconnected=off
  wires:
  Subtract/1 -> MATLAB Function/1(u)
  Constant/1 -> MATLAB Function/2(t_prp2)
  MATLAB Function/1(flag_base_drag) -> flag_base_drag/1  "flag_base_drag"
  Bus Selector1/1 -> Subtract/1  "<T_sim_glbl>"
  Bus Selector1/2 -> Subtract/2  "<T_sim_lnch>"
  env_glbl/1 -> Bus Selector1/1

== system PILnewH/Non-linear Flight Dynamic Model/Subsystem1/GRM_Airframe/environment/WGS84_Gravitation ==
  lon : Inport  PortDimensions=1
  lat : Inport  Port=2  PortDimensions=1
  h : Inport  Port=3  PortDimensions=1
  Assertion : Assertion  AssertionFailFcn="error('WGS84 Gravitationsmodell: Die Werte des Eingangs \"h\" muessen groesser als 0 sein')"
  Assertion1 : Assertion  AssertionFailFcn="error('WGS84 Gravitationsmodell: Die Werte des Eingangs \"Long\" muessen zwischen -180 und +180 liegen')"
  Assertion2 : Assertion  AssertionFailFcn="error('WGS84 Gravitationsmodell: Die Werte des Eingangs \"Lat\" muessen zwischen -90 und +90 liegen')"
  Compare To Constant : simulink/Logic and Bit Operations/Compare To Constant  relop=>=  const=0  OutDataTypeStr=boolean
      settings: SourceProductName=ISim Simulink Block Set
  Interval Test : simulink/Logic and Bit Operations/Interval Test  IntervalClosedRight=on  uplimit=pi  IntervalClosedLeft=on  lowlimit=-pi  OutDataTypeStr=boolean
      settings: SourceProductName=ISim Simulink Block Set
  Interval Test1 : simulink/Logic and Bit Operations/Interval Test  IntervalClosedRight=on  uplimit=pi/2  IntervalClosedLeft=on  lowlimit=-pi/2  OutDataTypeStr=boolean
      settings: SourceProductName=ISim Simulink Block Set
  WGS84_2_ECEF : Subsystem
  WGS84_Gravity_Implementation : MATLAB Function  TreatAsAtomicUnit=on
  gE : Outport  PortDimensions=3  VectorParamsAs1DForOutWhenUnconnected=off
  wires:
  Interval Test1/1 -> Assertion2/1
  Interval Test/1 -> Assertion1/1
  Compare To Constant/1 -> Assertion/1
  WGS84_2_ECEF/1(pE) -> WGS84_Gravity_Implementation/1(pE)  "pE"
  lat/1 -> WGS84_Gravity_Implementation/2(lat_rad), Interval Test1/1, WGS84_2_ECEF/3(lat)  "lat"
  lon/1 -> WGS84_Gravity_Implementation/3(long_rad), Interval Test/1, WGS84_2_ECEF/2(lon)  "lon"
  h/1 -> WGS84_2_ECEF/1(h), Compare To Constant/1  "h"
  WGS84_Gravity_Implementation/1(gamma_R) -> gE/1  "gE"

== system PILnewH/Non-linear Flight Dynamic Model/Subsystem1/GRM_Airframe/environment/atmosphere_static_ISO_2533 ==
  hBE : Inport
  env_glbl : Inport  Port=2
  Bus Creator1 : BusCreator  Inputs=6
  Bus Selector1 : BusSelector  OutputSignals=e_Tmp,e_pa
  Saturation : Saturate  UpperLimit=c_h_geope  LowerLimit=c_h_geop0
      settings: AttributesFormatString=|
      | %<UpperLimit>
      | %<LowerLimit>
  density : Subsystem
  geopot_height : Subsystem  mask{mean_earth_radius=c_r0}
      mask prompts: mean_earth_radius "Mean Earth Radius WGS 84 [m]"
      mask TypeOptions mean_earth_radius: mean_earth_radius/Value
  speed_of_sound : Subsystem
  tmp_and_pressure_ISO_2533 : Subsystem
  atm_stat : Outport  VectorParamsAs1DForOutWhenUnconnected=off
  wires:
  speed_of_sound/1(sos) -> Bus Creator1/3
  env_glbl/1 -> Bus Selector1/1
  Bus Selector1/2 -> tmp_and_pressure_ISO_2533/3(e_pa)  "<e_pa>"
  geopot_height/1(h_geop) -> Saturation/1
  Bus Selector1/1 -> tmp_and_pressure_ISO_2533/2(e_Tmp)  "<e_Tmp>"
  Bus Creator1/1 -> atm_stat/1  "atm_stat_bus"
  tmp_and_pressure_ISO_2533/1(Tmp) -> speed_of_sound/1(Tmp), Bus Creator1/4, density/1(Tmp)
  tmp_and_pressure_ISO_2533/2(pa) -> Bus Creator1/6, density/2(pa)
  density/1(rho) -> Bus Creator1/5
  hBE/1 -> Bus Creator1/1, geopot_height/1(hBE)
  Saturation/1 -> Bus Creator1/2, tmp_and_pressure_ISO_2533/1(h_geop)  "h_geop"

== system PILnewH/Non-linear Flight Dynamic Model/Subsystem1/GRM_Airframe/environment/convert_to_local_frame ==
  gE : Inport
  Constant1 : Constant  Value=0
  Dot Product : DotProduct  InputSameDT=on  OutDataTypeStr=Inherit: Inherit via internal rule
  Sqrt : Sqrt  SaturateOnIntegerOverflow=on
  Vector Concatenate : Concatenate  NumInputs=3  Mode=Multidimensional array
  gBG : Outport  VectorParamsAs1DForOutWhenUnconnected=off
  wires:
  gE/1 -> Dot Product/1, Dot Product/2
  Constant1/1 -> Vector Concatenate/2, Vector Concatenate/1
  Sqrt/1 -> Vector Concatenate/3
  Vector Concatenate/1 -> gBG/1  "gBG"
  Dot Product/1 -> Sqrt/1

== system PILnewH/Non-linear Flight Dynamic Model/Subsystem1/GRM_Airframe/fin_actuators/Rudder ==
  siB_c : Inport
  tRRR : Inport  Port=2
  Add : Sum  Inputs=+-
  Add1 : Sum  Inputs=+-
  Add2 : Sum  Inputs=+++
  Constant1 : Constant  Value=Actuator.fin1_bias
      settings: AttributesFormatString=%<Value>
  Gain : Gain  Gain=omega^2
  Gain2 : Gain  Gain=2*dmp*omega  Multiplication=Matrix(K*u)
  Gain3 : Gain  Gain=unc_bl
  Gain4 : Gain  Gain=Actuator.fin1_scale
      settings: AttributesFormatString=%<Gain>
  Integrator : Integrator  ExternalReset=either  InitialCondition=d_siB_0
  Integrator1 : Integrator  InitialCondition=siB_0  LimitOutput=on  UpperSaturationLimit=siB_max  LowerSaturationLimit=siB_min  ShowSaturationPort=on
  Limiting_Acceleration : MATLAB Function  TreatAsAtomicUnit=on
  Limiting_Rate : MATLAB Function  TreatAsAtomicUnit=on
  Saturation : Saturate  UpperLimit=siB_max  LowerLimit=siB_min
  Saturation1 : Saturate  UpperLimit=siB_max  LowerLimit=siB_min
  Sign : Signum
  siB : Outport  VectorParamsAs1DForOutWhenUnconnected=off
  d_siB : Outport  Port=2  VectorParamsAs1DForOutWhenUnconnected=off
  dd_siB : Outport  Port=3  VectorParamsAs1DForOutWhenUnconnected=off
  wires:
  Saturation1/1 -> siB/1, [siB]  "siB"
  Integrator1/2 -> Integrator/2  "sat"
  Gain4/1 -> Add2/2
  Gain3/1 -> Add2/3
  Sign/1 -> Gain3/1
  tRRR/1 -> Sign/1  "tRRR"
  Integrator1/1 -> Gain4/1, Add/2  "siB"
  Add1/1 -> Limiting_Acceleration/3(dd_siB)  "dd_siB"
  Gain2/1 -> Add1/2
  Gain/1 -> Add1/1
  Add/1 -> Gain/1
  Limiting_Acceleration/1(dd_siB_l) -> Integrator/1, dd_siB/1  "dd_siB_l"
  Limiting_Rate/1(d_siB_l) -> d_siB/1, [d_siB], Integrator1/1  "d_siB_l"
  Integrator/1 -> Limiting_Rate/2(d_siB), Gain2/1  "d_siB"
  Saturation/1 -> Add/1
  Add2/1 -> Saturation1/1
  Constant1/1 -> Add2/1
  siB_c/1 -> Saturation/1  "siB_c"
  [d_siB] -> Limiting_Acceleration/2(d_siB)
  [siB] -> Limiting_Acceleration/1(siB)
  [siB] -> Limiting_Rate/1(siB)

== system PILnewH/Non-linear Flight Dynamic Model/Subsystem1/GRM_Airframe/fin_actuators/Rudder1 ==
  siB_c : Inport
  tRRR : Inport  Port=2
  Add : Sum  Inputs=+-
  Add1 : Sum  Inputs=+-
  Add3 : Sum  Inputs=+++
  Constant1 : Constant  Value=Actuator.fin2_bias
      settings: AttributesFormatString=%<Value>
  Gain : Gain  Gain=omega^2
  Gain2 : Gain  Gain=2*dmp*omega  Multiplication=Matrix(K*u)
  Gain3 : Gain  Gain=unc_bl
  Gain4 : Gain  Gain=Actuator.fin2_scale
      settings: AttributesFormatString=%<Gain>
  Integrator : Integrator  ExternalReset=either  InitialCondition=d_siB_0
  Integrator1 : Integrator  InitialCondition=siB_0  LimitOutput=on  UpperSaturationLimit=siB_max  LowerSaturationLimit=siB_min  ShowSaturationPort=on
  Limiting_Acceleration : MATLAB Function  TreatAsAtomicUnit=on
  Limiting_Rate : MATLAB Function  TreatAsAtomicUnit=on
  Saturation : Saturate  UpperLimit=siB_max  LowerLimit=siB_min
  Saturation1 : Saturate  UpperLimit=siB_max  LowerLimit=siB_min
  Sign : Signum
  siB : Outport  VectorParamsAs1DForOutWhenUnconnected=off
  d_siB : Outport  Port=2  VectorParamsAs1DForOutWhenUnconnected=off
  dd_siB : Outport  Port=3  VectorParamsAs1DForOutWhenUnconnected=off
  wires:
  Saturation1/1 -> siB/1, [siB]  "siB"
  Integrator1/2 -> Integrator/2  "sat"
  Gain3/1 -> Add3/3
  Sign/1 -> Gain3/1
  tRRR/1 -> Sign/1  "tRRR"
  Integrator1/1 -> Add/2, Gain4/1  "siB"
  Add1/1 -> Limiting_Acceleration/3(dd_siB)  "dd_siB"
  Gain2/1 -> Add1/2
  Gain/1 -> Add1/1
  Add/1 -> Gain/1
  Limiting_Acceleration/1(dd_siB_l) -> Integrator/1, dd_siB/1  "dd_siB_l"
  Limiting_Rate/1(d_siB_l) -> d_siB/1, [d_siB], Integrator1/1  "d_siB_l"
  Integrator/1 -> Limiting_Rate/2(d_siB), Gain2/1  "d_siB"
  Saturation/1 -> Add/1
  Add3/1 -> Saturation1/1
  siB_c/1 -> Saturation/1  "siB_c"
  [d_siB] -> Limiting_Acceleration/2(d_siB)
  [siB] -> Limiting_Acceleration/1(siB)
  [siB] -> Limiting_Rate/1(siB)
  Constant1/1 -> Add3/1
  Gain4/1 -> Add3/2

== system PILnewH/Non-linear Flight Dynamic Model/Subsystem1/GRM_Airframe/fin_actuators/Rudder2 ==
  siB_c : Inport
  tRRR : Inport  Port=2
  Add : Sum  Inputs=+-
  Add1 : Sum  Inputs=+-
  Add3 : Sum  Inputs=+++
  Constant1 : Constant  Value=Actuator.fin3_bias
      settings: AttributesFormatString=%<Value>
  Gain : Gain  Gain=omega^2
  Gain2 : Gain  Gain=2*dmp*omega  Multiplication=Matrix(K*u)
  Gain3 : Gain  Gain=unc_bl
  Gain4 : Gain  Gain=Actuator.fin3_scale
      settings: AttributesFormatString=%<Gain>
  Integrator : Integrator  ExternalReset=either  InitialCondition=d_siB_0
  Integrator1 : Integrator  InitialCondition=siB_0  LimitOutput=on  UpperSaturationLimit=siB_max  LowerSaturationLimit=siB_min  ShowSaturationPort=on
  Limiting_Acceleration : MATLAB Function  TreatAsAtomicUnit=on
  Limiting_Rate : MATLAB Function  TreatAsAtomicUnit=on
  Saturation : Saturate  UpperLimit=siB_max  LowerLimit=siB_min
  Saturation1 : Saturate  UpperLimit=siB_max  LowerLimit=siB_min
  Sign : Signum
  siB : Outport  VectorParamsAs1DForOutWhenUnconnected=off
  d_siB : Outport  Port=2  VectorParamsAs1DForOutWhenUnconnected=off
  dd_siB : Outport  Port=3  VectorParamsAs1DForOutWhenUnconnected=off
  wires:
  Saturation1/1 -> siB/1, [siB]  "siB"
  Integrator1/2 -> Integrator/2  "sat"
  Gain3/1 -> Add3/3
  Sign/1 -> Gain3/1
  tRRR/1 -> Sign/1  "tRRR"
  Integrator1/1 -> Gain4/1, Add/2  "siB"
  Add1/1 -> Limiting_Acceleration/3(dd_siB)  "dd_siB"
  Gain2/1 -> Add1/2
  Gain/1 -> Add1/1
  Add/1 -> Gain/1
  Limiting_Acceleration/1(dd_siB_l) -> Integrator/1, dd_siB/1  "dd_siB_l"
  Limiting_Rate/1(d_siB_l) -> d_siB/1, [d_siB], Integrator1/1  "d_siB_l"
  Integrator/1 -> Limiting_Rate/2(d_siB), Gain2/1  "d_siB"
  Saturation/1 -> Add/1
  Add3/1 -> Saturation1/1
  siB_c/1 -> Saturation/1  "siB_c"
  [d_siB] -> Limiting_Acceleration/2(d_siB)
  [siB] -> Limiting_Acceleration/1(siB)
  [siB] -> Limiting_Rate/1(siB)
  Constant1/1 -> Add3/1
  Gain4/1 -> Add3/2

== system PILnewH/Non-linear Flight Dynamic Model/Subsystem1/GRM_Airframe/fin_actuators/Rudder3 ==
  siB_c : Inport
  tRRR : Inport  Port=2
  Add : Sum  Inputs=+-
  Add1 : Sum  Inputs=+-
  Add3 : Sum  Inputs=+++
  Constant1 : Constant  Value=Actuator.fin4_bias
      settings: AttributesFormatString=%<Value>
  Gain : Gain  Gain=omega^2
  Gain2 : Gain  Gain=2*dmp*omega  Multiplication=Matrix(K*u)
  Gain3 : Gain  Gain=unc_bl
  Gain4 : Gain  Gain=Actuator.fin4_scale
      settings: AttributesFormatString=%<Gain>
  Integrator : Integrator  ExternalReset=either  InitialCondition=d_siB_0
  Integrator1 : Integrator  InitialCondition=siB_0  LimitOutput=on  UpperSaturationLimit=siB_max  LowerSaturationLimit=siB_min  ShowSaturationPort=on
  Limiting_Acceleration : MATLAB Function  TreatAsAtomicUnit=on
  Limiting_Rate : MATLAB Function  TreatAsAtomicUnit=on
  Saturation : Saturate  UpperLimit=siB_max  LowerLimit=siB_min
  Saturation1 : Saturate  UpperLimit=siB_max  LowerLimit=siB_min
  Sign : Signum
  siB : Outport  VectorParamsAs1DForOutWhenUnconnected=off
  d_siB : Outport  Port=2  VectorParamsAs1DForOutWhenUnconnected=off
  dd_siB : Outport  Port=3  VectorParamsAs1DForOutWhenUnconnected=off
  wires:
  Saturation1/1 -> siB/1, [siB]  "siB"
  Integrator1/2 -> Integrator/2  "sat"
  Gain3/1 -> Add3/3
  Sign/1 -> Gain3/1
  tRRR/1 -> Sign/1  "tRRR"
  Integrator1/1 -> Gain4/1, Add/2  "siB"
  Add1/1 -> Limiting_Acceleration/3(dd_siB)  "dd_siB"
  Gain2/1 -> Add1/2
  Gain/1 -> Add1/1
  Add/1 -> Gain/1
  Limiting_Acceleration/1(dd_siB_l) -> Integrator/1, dd_siB/1  "dd_siB_l"
  Limiting_Rate/1(d_siB_l) -> d_siB/1, [d_siB], Integrator1/1  "d_siB_l"
  Integrator/1 -> Limiting_Rate/2(d_siB), Gain2/1  "d_siB"
  Saturation/1 -> Add/1
  Add3/1 -> Saturation1/1
  siB_c/1 -> Saturation/1  "siB_c"
  [d_siB] -> Limiting_Acceleration/2(d_siB)
  [siB] -> Limiting_Acceleration/1(siB)
  [siB] -> Limiting_Rate/1(siB)
  Constant1/1 -> Add3/1
  Gain4/1 -> Add3/2

== system PILnewH/Non-linear Flight Dynamic Model/Subsystem1/GRM_Airframe/fin_actuators/control_allocation ==
  siB : Inport
  d_siB : Inport  Port=2
  dd_siB : Inport  Port=3
  Constant8 : Constant  Value=Tr3r4
  Product : Product  Multiplication=Matrix(*)
  Product1 : Product  Multiplication=Matrix(*)
  Product2 : Product  Multiplication=Matrix(*)
  Tr3r4 : Outport  VectorParamsAs1DForOutWhenUnconnected=off
  finB : Outport  Port=2  VectorParamsAs1DForOutWhenUnconnected=off
  d_finB : Outport  Port=3  VectorParamsAs1DForOutWhenUnconnected=off
  dd_finB : Outport  Port=4  VectorParamsAs1DForOutWhenUnconnected=off
  wires:
  Product/1 -> finB/1  "afinB"
  Constant8/1 -> Tr3r4/1, Product2/1, Product1/1, Product/1  "Tr3r4"
  siB/1 -> Product/2
  d_siB/1 -> Product1/2
  Product1/1 -> d_finB/1  "d_afinB"
  dd_siB/1 -> Product2/2
  Product2/1 -> dd_finB/1  "dd_afinB"
